simulink model "square_pulse_baseband"  (R2023b)
settings: Solver=VariableStepAuto  StartTime=0.0  StopTime=10000  RelTol=1e-3
InitFcn:
  | bps = 1;
  | res = 50;
undefined symbols (not defined in the file): DiscIntNeverNeededParam
libraries: commchan3 x1, commrandsrc3 x1, commfilt2 x1
settings Model: PauseTimes=4  Creator=hchintak  LastModifiedBy=Harish

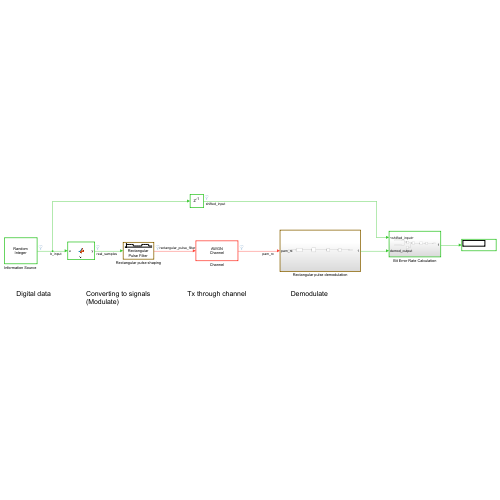
[thumbnail: Simulink's stored preview of the top-level diagram]
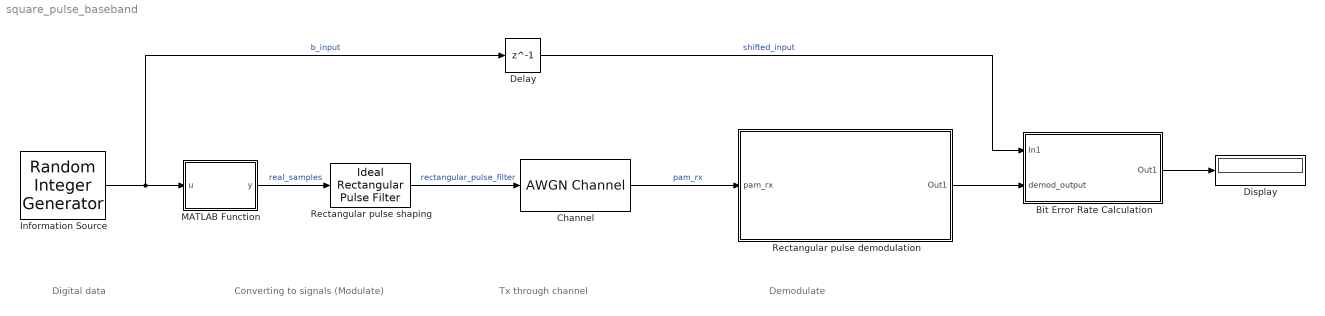
== system square_pulse_baseband ==
  note: Tx through channel
  note: Converting to signals
      | (Modulate)
  note: Digital data
  note: Demodulate
  Bit Error Rate Calculation : Subsystem
  Channel : commchan3/AWGN Channel  LegacyMode=off  NoiseMethod="Signal to noise ratio  (Eb/No)"  noiseMode="Signal to noise ratio  (SNR)"  EbNo=0  EsNo=10  SNR=10  BitsPerSymbol=1  SignalPower=1  SamplesPerSymbol=res  SymbolPeriod=1  VarianceSource=Parameter  Variance=1  RandomStream=Global stream  Seed=67  SimulateUsing=Code generation
  Delay : Delay  DelayLength=1
  Display : Display
  "Information Source " : commrandsrc3/Random Integer Generator  SetSize=2  SeedSource=Auto  Seed=0  SampleTime=bps  SamplesPerFrame=1  OutputDataType=double  SimulateUsing=Interpreted execution
  MATLAB Function : MATLAB Function  TreatAsAtomicUnit=on
  Rectangular pulse demodulation : Subsystem
  Rectangular pulse shaping : commfilt2/Ideal Rectangular Pulse Filter  pulseLen=res  pulseDelay=0  InputProcessing=Columns as channels (frame based)  RateOptions=Allow multirate processing  sampMode=Mute  normCheck=off  normMode=Sum of samples  filterGain=1  saveAsFlag=0  roundingMode=Floor  overflowMode=off  firstCoeffDataTypeStr=Inherit: Same word length as input  firstCoeffMin=[]  firstCoeffMax=[]  firstCoeffLastDataTypeStr=Inherit: Same word length as input  outputDataTypeStr=Inherit: Same as accumulator  outputMin=[]  outputMax=[]  outputLastDataTypeStr=Inherit: Same as accumulator
  wires:
  "Information Source "/1 -> MATLAB Function/1(u), Delay/1  "b_input"
  Rectangular pulse shaping/1 -> Channel/1  "rectangular_pulse_filter"
  Bit Error Rate Calculation/1(Out1) -> Display/1
  Delay/1 -> Bit Error Rate Calculation/1(In1)  "shifted_input"
  MATLAB Function/1(y) -> Rectangular pulse shaping/1  "real_samples"
  Channel/1 -> Rectangular pulse demodulation/1(pam_rx)  "pam_rx"
  Rectangular pulse demodulation/1(Out1) -> Bit Error Rate Calculation/2(demod_output)

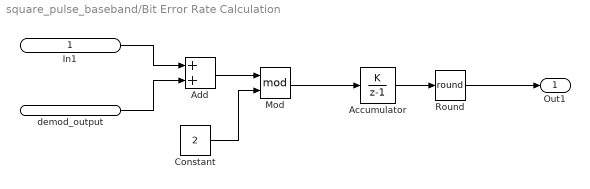
== system square_pulse_baseband/Bit Error Rate Calculation ==
  In1 : Inport
  demod_output : Inport  Port=2
  Accumulator : DiscreteIntegrator  IntegratorMethod=Accumulation: Forward Euler  SampleTime=-1  ICPrevOutput=DiscIntNeverNeededParam  ICPrevScaledInput=DiscIntNeverNeededParam
  Add : Sum
  Constant : Constant  Value=2
  Mod : Math  Operator=mod
  Round : Rounding  Operator=round
  Out1 : Outport
  wires:
  Accumulator/1 -> Round/1
  In1/1 -> Add/1
  demod_output/1 -> Add/2
  Add/1 -> Mod/1
  Constant/1 -> Mod/2
  Mod/1 -> Accumulator/1
  Round/1 -> Out1/1

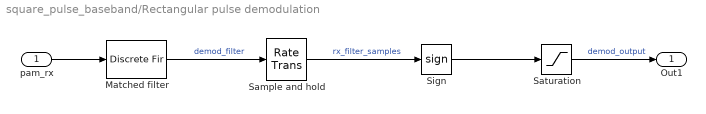
== system square_pulse_baseband/Rectangular pulse demodulation ==
  pam_rx : Inport
  Matched filter : DiscreteFir  Coefficients=(1/res)*[0,ones(1,res)]
  Sample and hold : RateTransition  Deterministic=off  OutPortSampleTime=bps
  Saturation : Saturate  UpperLimit=1  LowerLimit=0
  Sign : Signum
  Out1 : Outport
  wires:
  Saturation/1 -> Out1/1  "demod_output"
  Sign/1 -> Saturation/1
  Matched filter/1 -> Sample and hold/1  "demod_filter"
  pam_rx/1 -> Matched filter/1
  Sample and hold/1 -> Sign/1  "rx_filter_samples"

== matlab function square_pulse_baseband/MATLAB Function ==
  data: u input; y output
function y = fcn(u)

y = 2*u-1;
